simulink model "state_func_val"  (R2022a)
settings: Solver=ode15s  StartTime=0.0  StopTime=5  MaxStep=0.01  RelTol=1e-3
values from neighbouring files (symbols this model uses):
  nx = 12 + 2*n    [nmpc_matlab.m]    (also in nmpc_test.m)
  ny = 8    [nmpc_matlab.m]    (also in nmpc_test.m)
  q0 = zeros(N, 1)    [ee_dyn_check.m]    (also in matrices_time_test.m = [0.1; 0.2; 0.3; pi/2; pi/2; pi/2])
  tau = [taub; taum]    [ee_dyn_check.m]
undefined symbols (not defined in the file or in its folder): fx, fy, fz, nz, q_dot0, xee0, xee_dot0
settings Model: Creator=charl  LastModifiedBy=charl

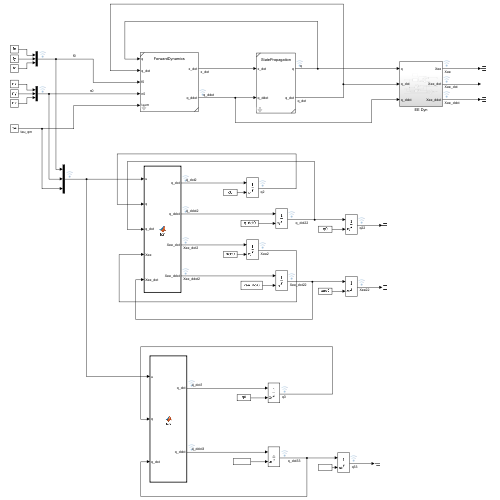
[thumbnail: Simulink's stored preview of the top-level diagram]
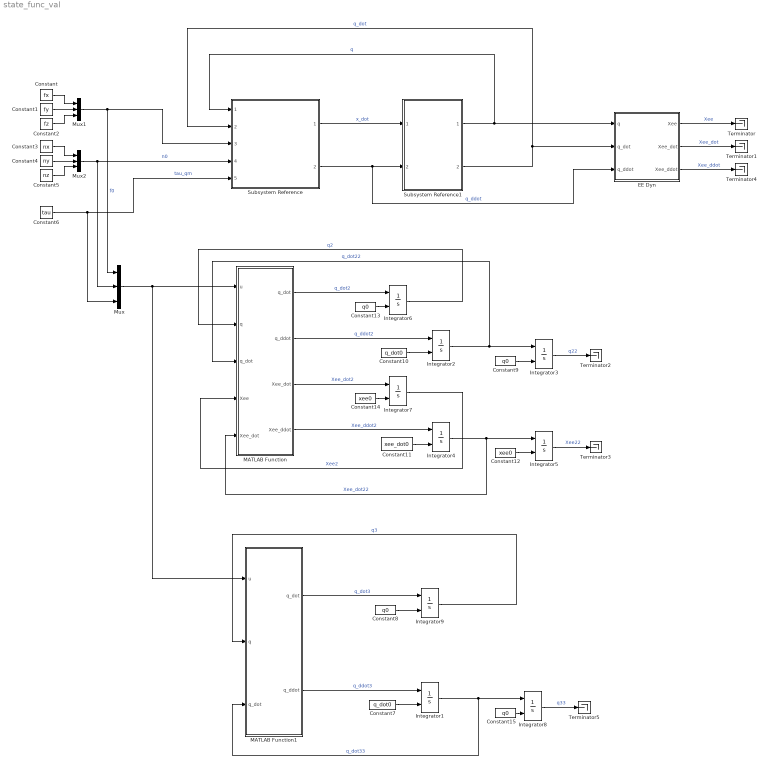
== system state_func_val ==
  Constant : Constant  Value=fx
  Constant1 : Constant  Value=fy
  Constant10 : Constant  Value=q_dot0
  Constant11 : Constant  Value=xee_dot0
  Constant12 : Constant  Value=xee0
  Constant{8..9,13,15} (4 alike) : Constant  Value=q0
  Constant14 : Constant  Value=xee0
  Constant2 : Constant  Value=fz
  Constant3 : Constant  Value=nx
  Constant4 : Constant  Value=ny
  Constant5 : Constant  Value=nz
  Constant6 : Constant  Value=tau
  Constant7 : Constant  Value=q_dot0
  EE Dyn : Subsystem
  Integrator{1..9} (9 alike) : Integrator  InitialConditionSource=external
  MATLAB Function : MATLAB Function  TreatAsAtomicUnit=on
  MATLAB Function1 : MATLAB Function  TreatAsAtomicUnit=on
  Mux : Mux  Inputs=3
  Mux1 : Mux  Inputs=3
  Mux2 : Mux  Inputs=3
  Subsystem Reference : Subsystem  ReferencedSubsystem=ForwardDynamics  spaceRobot=sr  SimulateUsing=Interpreted execution
  Subsystem Reference1 : Subsystem  ReferencedSubsystem=StatePropagation  spaceRobot=sr  q_0=q0  q_dot_0=q_dot0
  Terminator{,1..5} (6 alike) : Terminator
  wires:
  Constant1/1 -> Mux1/2
  Constant9/1 -> Integrator3/2
  Constant6/1 -> Mux/3, Subsystem Reference/5  "tau_qm"
  MATLAB Function/2(q_ddot) -> Integrator2/1  "q_ddot2"
  Constant4/1 -> Mux2/2
  Mux1/1 -> Mux/1, Subsystem Reference/3  "f0"
  Integrator2/1 -> MATLAB Function/3("q_dot "), Integrator3/1  "q_dot22"
  Mux2/1 -> Mux/2, Subsystem Reference/4  "n0"
  Constant2/1 -> Mux1/3
  Constant5/1 -> Mux2/3
  Constant10/1 -> Integrator2/2
  Constant3/1 -> Mux2/1
  Constant/1 -> Mux1/1
  EE Dyn/1(Xee) -> Terminator/1  "Xee"
  EE Dyn/2(Xee_dot) -> Terminator1/1  "Xee_dot"
  Constant11/1 -> Integrator4/2
  MATLAB Function/4(Xee_ddot) -> Integrator4/1  "Xee_ddot2"
  Integrator4/1 -> MATLAB Function/5("Xee_dot "), Integrator5/1  "Xee_dot22"
  Constant12/1 -> Integrator5/2
  MATLAB Function/1(q_dot) -> Integrator6/1  "q_dot2"
  Constant13/1 -> Integrator6/2
  Integrator6/1 -> MATLAB Function/2(q)  "q2"
  Integrator3/1 -> Terminator2/1  "q22"
  Constant14/1 -> Integrator7/2
  MATLAB Function/3(Xee_dot) -> Integrator7/1  "Xee_dot2"
  Integrator7/1 -> MATLAB Function/4(Xee)  "Xee2"
  Integrator5/1 -> Terminator3/1  "Xee22"
  EE Dyn/3(Xee_ddot) -> Terminator4/1  "Xee_ddot"
  Subsystem Reference/2 -> EE Dyn/3(q_ddot), Subsystem Reference1/2  "q_ddot"
  Subsystem Reference1/1 -> Subsystem Reference/1, EE Dyn/1(q)  "q"
  Subsystem Reference1/2 -> Subsystem Reference/2, EE Dyn/2(q_dot)  "q_dot"
  Mux/1 -> MATLAB Function1/1(u), MATLAB Function/1(u)
  Integrator9/1 -> MATLAB Function1/2(q)  "q3"
  Integrator8/1 -> Terminator5/1  "q33"
  Constant8/1 -> Integrator9/2
  MATLAB Function1/2(q_ddot) -> Integrator1/1  "q_ddot3"
  MATLAB Function1/1(q_dot) -> Integrator9/1  "q_dot3"
  Constant7/1 -> Integrator1/2
  Integrator1/1 -> MATLAB Function1/3("q_dot "), Integrator8/1  "q_dot33"
  Constant15/1 -> Integrator8/2
  Subsystem Reference/1 -> Subsystem Reference1/1  "x_dot"

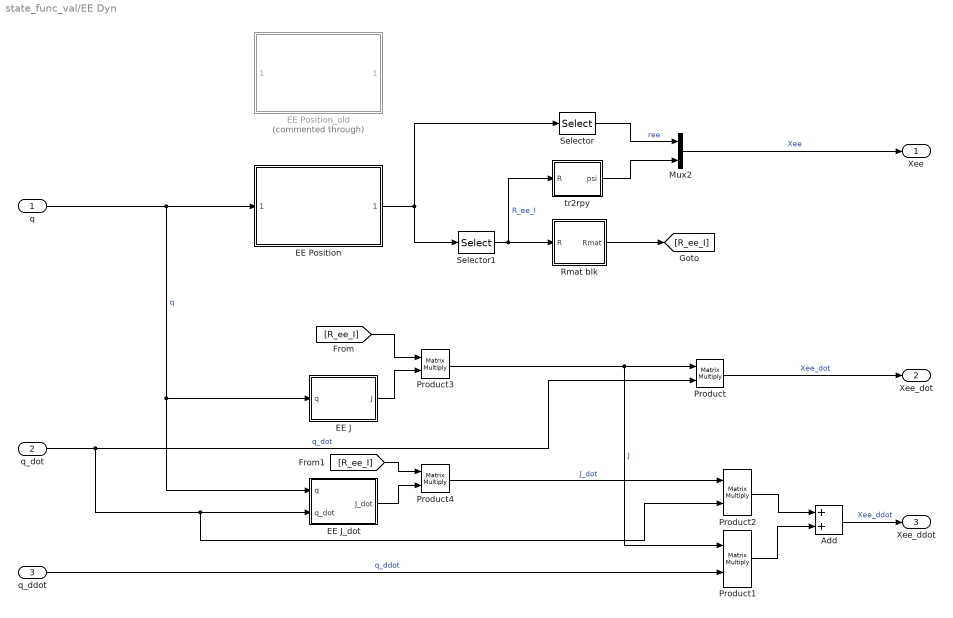
== system state_func_val/EE Dyn ==
  q : Inport
  q_dot : Inport  Port=2
  q_ddot : Inport  Port=3
  Add : Sum
  EE J : MATLAB Function  TreatAsAtomicUnit=on
  EE J_dot : MATLAB Function  TreatAsAtomicUnit=on
  EE Position : Subsystem  ReferencedSubsystem=GetTransformEE  spaceRobot=sr
  EE Position_old : Subsystem  Commented=through  ReferencedSubsystem=GetTransform  spaceRobot=sr  sourceBody=endeffector  targetBody=inertial  SimulateUsing=Interpreted execution
  Mux2 : Mux  Inputs=2
  Product{,1..4} (5 alike) : Product  Multiplication=Matrix(*)
  Rmat blk : MATLAB Function  TreatAsAtomicUnit=on
  Selector : Selector  NumberOfDimensions=2  InputPortWidth=[4 4]  IndexOptions=Index vector (dialog),Index vector (dialog)  Indices=[1:3],4  OutputSizes=1,1
  Selector1 : Selector  NumberOfDimensions=2  InputPortWidth=[4 4]  IndexOptions=Index vector (dialog),Index vector (dialog)  Indices=[1:3],[1:3]  OutputSizes=1,1
  tr2rpy : MATLAB Function  TreatAsAtomicUnit=on
  Xee : Outport
  Xee_dot : Outport  Port=2
  Xee_ddot : Outport  Port=3
  wires:
  Selector1/1 -> tr2rpy/1(R), Rmat blk/1(R)  "R_ee_I"
  Product3/1 -> Product/1, Product1/1  "J"
  q_dot/1 -> Product/2, Product2/2, EE J_dot/2(q_dot)  "q_dot"
  EE J/1(J) -> Product3/2
  [R_ee_I] -> Product3/1
  Product2/1 -> Add/1
  EE Position/1 -> Selector/1, Selector1/1
  q/1 -> EE Position/1, EE J_dot/1(q), EE J/1(q)  "q"
  Product1/1 -> Add/2
  Selector/1 -> Mux2/1  "ree"
  Product4/1 -> Product2/1  "J_dot"
  Rmat blk/1(Rmat) -> [R_ee_I]
  EE J_dot/1(J_dot) -> Product4/2
  Add/1 -> Xee_ddot/1  "Xee_ddot"
  Product/1 -> Xee_dot/1  "Xee_dot"
  [R_ee_I] -> Product4/1
  q_ddot/1 -> Product1/2  "q_ddot"
  tr2rpy/1(psi) -> Mux2/2
  Mux2/1 -> Xee/1  "Xee"

== matlab function state_func_val/MATLAB Function ==
  data: u input; q_dot output; q input; q_ddot output; Xee_dot output; q_dot input; Xee input; Xee_dot input; Xee_ddot output
function [q_dot, q_ddot, Xee_dot, Xee_ddot] = fcn(u, q, q_dot, Xee, Xee_dot)

x = [q; Xee; q_dot; Xee_dot];


dx = sr_ee_state_func(x, u);

q_dot = dx(1:8);
q_ddot = dx(15:22);

Xee_dot = dx(9:14);
Xee_ddot = dx(23:28);

== matlab function state_func_val/EE Dyn/EE J ==
  data: q input; J output
function J = fcn(q)
sr_info = SR2_info();

% 1 - Kinematics
[Rb, Ra, Rm] = RFunc_SR2(q);
Rm = reshape(Rm, 3, 3, []); % Split Rm to nk 3x3 arrays

% 2 - Kinetics
[~, ~, ~, A, ~] = Kin(sr_info, q, zeros(8, 1), zeros(8, 1), {Rb, Ra, Rm});

% 3 - J
J = Jacobian('endeffector', sr_info, A, {Rb, Ra});

% J_dot = Jacobian_dot('endeffector', sr_info, A, A_dot, {Rb, Ra}, wb, Omega);

end

== matlab function state_func_val/EE Dyn/EE J_dot ==
  data: q input; J_dot output; q_dot input
function J_dot = fcn(q, q_dot)
sr_info = SR2_info();

% 1 - Kinematics
[Rb, Ra, Rm] = RFunc_SR2(q);
Rm = reshape(Rm, 3, 3, []); % Split Rm to nk 3x3 arrays

% 2 - Kinetics
[t, ~, Omega, A, A_dot] = Kin(sr_info, q, q_dot, zeros(8, 1), {Rb, Ra, Rm});
wb = t{1}(4:6);

% 3 - J_dot
J_dot = Jacobian_dot('endeffector', sr_info, A, A_dot, {Rb, Ra}, wb, Omega);

== matlab function state_func_val/EE Dyn/Rmat blk ==
  data: R input; Rmat output
function Rmat = fcn(R)

Rmat = blkdiag(R, R);

== matlab function state_func_val/EE Dyn/tr2rpy ==
  data: R input; psi output size=[3, 1]
function psi = fcn(R)
% Computes euler angle from rotation matrix

psi = zeros(3, 1);

temp = rotm2eul(R, 'ZYX');
psi(1) = temp(3);
psi(2) = temp(2);
psi(3) = temp(1);

== matlab function state_func_val/MATLAB Function1 ==
  data: u input; q_dot output; q input; q_ddot output; q_dot input
function [q_dot, q_ddot] = fcn(u, q, q_dot)

x = [q; q_dot];


dx = sr_state_func(x, u);

q_dot = dx(1:8);
q_ddot = dx(9:16);
